simulink model "Amradio"  (Simulink 9.3)
settings: Solver=ode3  StartTime=0.0  StopTime=10.0  RelTol=1e-3
settings Model: Creator=vibhuti  LastModifiedBy=vibhuti
settings DataIOCC: SaveFormat=Dataset  SignalLoggingSaveFormat=Dataset  ReturnWorkspaceOutputs=on
settings OptimizationCC: LifeSpan=auto
settings DebuggingCC: UnderspecifiedInitializationDetection=Simplified  MergeDetectMultiDrivingBlocksExec=error  FcnCallInpInsideContextMsg=error  SFUnexpectedBacktrackingDiag=error  SFNoUnconditionalDefaultTransitionDiag=error  SFExecutionAtInitializationDiag=warning  ArithmeticOperatorsInVariantConditions=error
settings HardwareCC: ProdBitPerPointer=64  ProdBitPerSizeT=64  ProdBitPerPtrDiffT=64  ProdLargestAtomicFloat=Float  ProdIntDivRoundTo=Zero  ProdEndianess=LittleEndian  ProdWordSize=64  ProdHWDeviceType=Intel->x86-64 (Windows64)
settings ModelReferenceCC: PropagateSignalLabelsOutOfModel=on
settings SFSimCC: SimUseLocalCustomCode=on
settings RTWCC: RTWUseLocalCustomCode=on
settings CodeAppCC: StateflowObjectComments=off
settings GRTTargetCC: TargetLangStandard=C99 (ISO)  CombineOutputUpdateFcns=on  GRTInterface=off
settings ConfigComp: CovMetricSettings=dwe  CovHtmlReporting=off  CovSaveCumulativeToWorkspaceVar=off  CovSaveSingleToWorkspaceVar=off  CovExternalEMLEnable=on

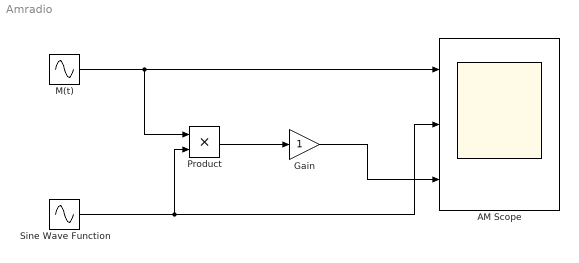
== system Amradio ==
  AM Scope : Scope  NumInputPorts=3
  Gain : Gain
  M(t) : Sin  Amplitude=2  Phase=pi/2  SampleTime=1/1000
  Product : Product
  Sine Wave Function : Sin  Frequency=25/(2*pi)  SampleTime=1/1000
  wires:
  M(t)/1 -> Product/1, AM Scope/1
  Sine Wave Function/1 -> Product/2, AM Scope/2
  Product/1 -> Gain/1
  Gain/1 -> AM Scope/3
